simulink model "Solar_system_sim"  (R2024b)
settings: Solver=VariableStepAuto  StartTime=0.0  StopTime=transfer_data.wait_time + transfer_data.T  MaxStep=1e4  RelTol=1e-6
values from neighbouring files (symbols this model uses):
  Earth = Solar_Orbit(R_earth,T_earth,deg2rad(51))    [Solar_system_setup.m]
  Mars = Solar_Orbit(R_mars,T_mars,deg2rad(143))    [Solar_system_setup.m]
  transfer_burn_time = 1    [Solar_system_setup.m]
  transfer_data = struct("wait_time", wait_time,                          "v_escape", v_escape,                          "v_encounter", v_encounter,                          "T", T)    [hohmann_transfer.m]
settings Model: Creator=cpero  LastModifiedBy=cpero

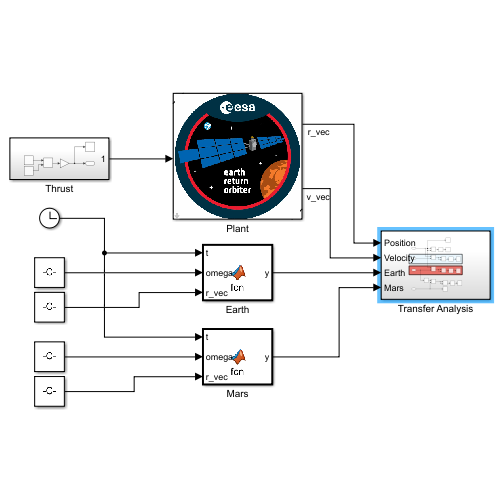
[thumbnail: Simulink's stored preview of the top-level diagram]
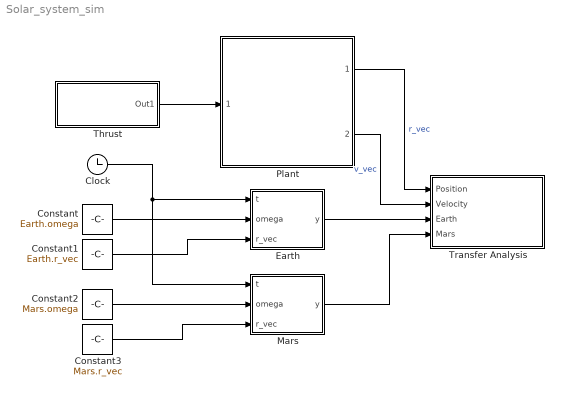
== system Solar_system_sim ==
  Clock : Clock
  Constant : Constant  Value=Earth.omega
  Constant1 : Constant  Value=Earth.r_vec
  Constant2 : Constant  Value=Mars.omega
  Constant3 : Constant  Value=Mars.r_vec
  Earth : MATLAB Function  TreatAsAtomicUnit=on
  Mars : MATLAB Function  TreatAsAtomicUnit=on
  Plant : Subsystem  ReferencedSubsystem=Plant  initial_data=transfer_initial  maneuver_time=transfer_data.wait_time  mu=Sun_mu
  Thrust : Subsystem
  Transfer Analysis : Subsystem
  wires:
  Clock/1 -> Mars/1(t), Earth/1(t)
  Constant/1 -> Earth/2(omega)
  Constant1/1 -> Earth/3(r_vec)
  Constant2/1 -> Mars/2(omega)
  Constant3/1 -> Mars/3(r_vec)
  Thrust/1(Out1) -> Plant/1
  Plant/1 -> Transfer Analysis/1(Position)  "r_vec"
  Plant/2 -> Transfer Analysis/2(Velocity)  "v_vec"
  Earth/1(y) -> Transfer Analysis/3(Earth)
  Mars/1(y) -> Transfer Analysis/4(Mars)

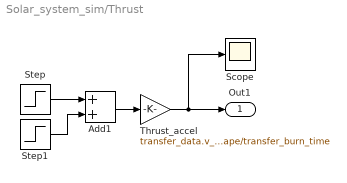
== system Solar_system_sim/Thrust ==
  Add1 : Sum
  Scope : Scope
  Step : Step  Time=transfer_data.wait_time  SampleTime=0
  Step1 : Step  Time=transfer_data.wait_time + transfer_burn_time  After=-1  SampleTime=0
  Thrust_accel : Gain  Gain=transfer_data.v_escape/transfer_burn_time
  Out1 : Outport
  wires:
  Add1/1 -> Thrust_accel/1
  Thrust_accel/1 -> Out1/1, Scope/1
  Step1/1 -> Add1/2
  Step/1 -> Add1/1

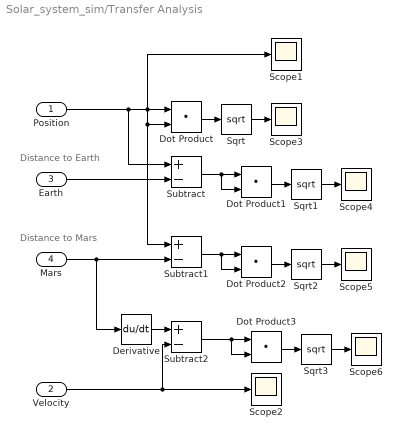
== system Solar_system_sim/Transfer Analysis ==
  note: Distance to Mars
  note: Distance to Earth
  Position : Inport
  Velocity : Inport  Port=2
  Earth : Inport  Port=3
  Mars : Inport  Port=4
  Derivative : Derivative
  Dot Product{,1..3} (4 alike) : DotProduct  OutDataTypeStr=Inherit: Inherit via internal rule
  Scope{1..6} (6 alike) : Scope
  Sqrt{,1..3} (4 alike) : Sqrt
  Subtract : Sum  Inputs=+-
  Subtract1 : Sum  Inputs=+-
  Subtract2 : Sum  Inputs=+-
  wires:
  Subtract1/1 -> Dot Product2/2, Dot Product2/1
  Dot Product2/1 -> Sqrt2/1
  Position/1 -> Scope1/1, Dot Product/2, Subtract1/1, Dot Product/1, Subtract/1
  Sqrt/1 -> Scope3/1
  Dot Product1/1 -> Sqrt1/1
  Sqrt2/1 -> Scope5/1
  Sqrt1/1 -> Scope4/1
  Dot Product/1 -> Sqrt/1
  Subtract/1 -> Dot Product1/2, Dot Product1/1
  Mars/1 -> Derivative/1, Subtract1/2
  Velocity/1 -> Subtract2/2, Scope2/1
  Earth/1 -> Subtract/2
  Derivative/1 -> Subtract2/1
  Sqrt3/1 -> Scope6/1
  Dot Product3/1 -> Sqrt3/1
  Subtract2/1 -> Dot Product3/2, Dot Product3/1

== matlab function Solar_system_sim/Mars ==
  data: t input; omega input; y output; r_vec input
function y = fcn(t, omega, r_vec)

rot_angle = omega*t;
rot = [cos(rot_angle), -sin(rot_angle), 0;
       sin(rot_angle), cos(rot_angle), 0;
       0, 0, 1];
y = rot*r_vec;

== matlab function Solar_system_sim/Earth ==
  data: t input; y output; omega input; r_vec input
function y = fcn(t, omega, r_vec)

rot_angle = omega*t;
rot = [cos(rot_angle), -sin(rot_angle), 0;
       sin(rot_angle), cos(rot_angle), 0;
       0, 0, 1];
y = rot*r_vec;
